simulink library "MicaServo"  (Simulink 4.00)
settings Model: LastModifiedBy=Administrator

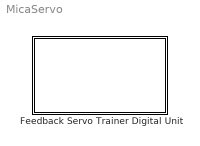
== system MicaServo ==
  Feedback Servo Trainer Digital Unit : Subsystem
      settings: RTWFcnNameOpts=Auto  RTWFileNameOpts=Auto
      mask Type: Feedback Servo Trainer Digital Unit with Mica926
      mask Display: disp ('Feedback 33-003 \n\n Digital Servo Fundementals \n with MICA 926')

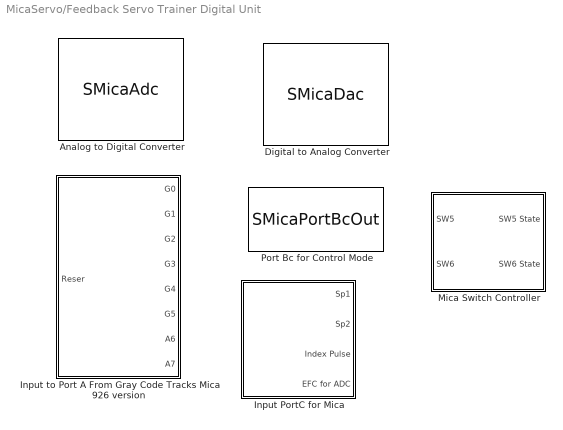
== system MicaServo/Feedback Servo Trainer Digital Unit ==
  " Digital to Analog Converter" : S-Function  FunctionName=SMicaDac  Parameters=baseAddr,inType,stime,hwAccess  PortCounts=[]  SFunctionModules=''  mask( Digital to Analog Converter){baseAddr=0x300, inType=RawData (-127 to +127), stime=0.01, hwAccess=on}
      mask prompts: baseAddr "BaseAddress"; inType "Input Type"; stime "Sampling Time (sec.)"; hwAccess "Access Hardware"
      mask help:
      | Analog Input Unit for Feedback DU154B
      | Digital Unit 33-003
      | Feeback Instruments
      | MICA 926 Edition
      mask Help:
      | Applies the corresponding voltage to the Servo Trainers DAC
      | output type can be selected to be either in RawData type or directly in volts
      mask StyleString: edit,popup(RawData (-127 to +127)| Volt   (+/- 11V range)),edit,checkbox
      mask Display: disp('Feedback Servo Trainer\n Digital Unit 33-003\n\n DAC\n Mica 926 Board ')
  Analog to Digital Converter : S-Function  FunctionName=SMicaAdc  Parameters=baseAddr,inType,stime,hwAccess  PortCounts=[]  SFunctionModules=''  mask(Analog to Digital Converter){baseAddr=0x300, inType=RawData (-127 to +127), stime=0.01, hwAccess=on}
      mask prompts: baseAddr "BaseAddress"; inType "Input Type"; stime "Sampling Time (sec.)"; hwAccess "Access Hardware"
      mask help:
      | Analog Input Unit for Feedback DU154B
      | Digital Unit 33-003
      | Feeback Instruments
      mask Help:
      | Reads and converts the voltage applied to ADC input on the Digital Unit.
      | Read operation is done either in Rawdata (+/- 127) format or directly in voltage format
      mask StyleString: edit,popup(RawData (-127 to +127)| Volt   (+/- 11V range)),edit,checkbox
      mask Display: disp('Feedback Servo Trainer\n Digital Unit 33-003\n\n ADC\n Mica 926 Board ')
  Input PortC for Mica : Subsystem  mask(Read the Inputs from portC directly){baseAddr=0x300, stime=0.01, hwAccess=on}
      mask prompts: baseAddr "BaseAddress"; stime "Sample Time (sec.)"; hwAccess "Access Hardware"
      settings: RTWFcnNameOpts=Auto  RTWFileNameOpts=Auto
  Input to Port A From Gray Code Tracks Mica 926 version : Subsystem  mask(Read Gray Code and Speed Tracks){baseAddr=0x300, stime=0.01, hwAccess=on}
      mask prompts: baseAddr "BaseAddress"; stime "Sample Time (sec.)"; hwAccess "Hardware Access"
      mask help:
      | Read the inputs from the Gray Code tracks (A0-A5)
      | and Speed/Increment tracks (A6-A7)
      settings: RTWFcnNameOpts=Auto  RTWFileNameOpts=Auto
      mask Help: no help is available for this block
  Mica Switch Controller : Subsystem  mask(Mica Switch Controller){baseAddr=0x300, onWhen=1.0, stime=0.01, hwAccess=on}
      mask prompts: baseAddr "BaseAddress"; onWhen "Thresh Hold"; stime "Sample Time (sec.)"; hwAccess "Hardware Access"
      mask help:
      | Controls the SW5 and SW6 switches on the Digital Unit
      | The ouptut can be used to see the state of the switches
      settings: RTWFcnNameOpts=Auto  RTWFileNameOpts=Auto
      mask Help: The Switches will be on when the input to the Swiches are bigger than or equal to the "Thresh Hold" variable
  Port Bc for Control Mode : S-Function  FunctionName=SMicaPortBcOut  Parameters=baseAddr,stime,hwAccess  PortCounts=[]  SFunctionModules=''  mask(Port Bc for Direct access to Control Signals){baseAddr=0x300, stime=0.01, hwAccess=on}
      mask prompts: baseAddr "Base Address"; stime "Sample Time (sec.)"; hwAccess "Access Hardware"
      mask help:
      | To directly access the Bc control register
      | For Advanced users only !
      mask Help:
      | Will directly apply the integer input to the Bc control output
      | This module is for advenced users only .
      | using this module with other Servo Trainer modules may corrupt inputs !
      mask Display: disp('Feedback Servo Trainer\n Digital Unit 33-003\n\nPort Bc \n Mica 926 Version')

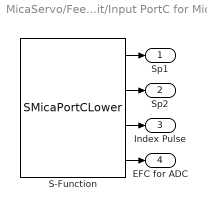
== system MicaServo/Feedback Servo Trainer Digital Unit/Input PortC for Mica ==
  S-Function : S-Function  FunctionName=SMicaPortCLower  Parameters=baseAddr,stime,hwAccess  PortCounts=[]  SFunctionModules=''
  Sp1 : Outport  Port=1
  Sp2 : Outport  Port=2
  Index Pulse : Outport  Port=3
  "EFC for ADC  " : Outport  Port=4
  wires:
  S-Function/4 -> "EFC for ADC  "/1
  S-Function/3 -> Index Pulse/1
  S-Function/2 -> Sp2/1
  S-Function/1 -> Sp1/1

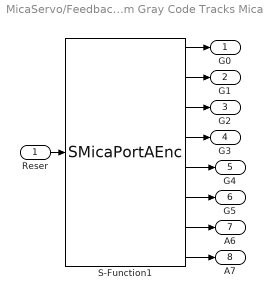
== system MicaServo/Feedback Servo Trainer Digital Unit/Input to Port A From Gray Code Tracks Mica 926 version ==
  Reser : Inport  Port=1
  S-Function1 : S-Function  FunctionName=SMicaPortAEnc  Parameters=baseAddr,stime,hwAccess  PortCounts=[]  SFunctionModules=''
  G0 : Outport  Port=1
  G1 : Outport  Port=2
  G2 : Outport  Port=3
  G3 : Outport  Port=4
  G4 : Outport  Port=5
  G5 : Outport  Port=6
  A6 : Outport  Port=7
  A7 : Outport  Port=8
  wires:
  S-Function1/8 -> A7/1
  S-Function1/7 -> A6/1
  S-Function1/6 -> G5/1
  S-Function1/5 -> G4/1
  Reser/1 -> S-Function1/1
  S-Function1/4 -> G3/1
  S-Function1/3 -> G2/1
  S-Function1/2 -> G1/1
  S-Function1/1 -> G0/1

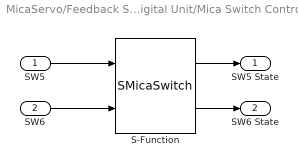
== system MicaServo/Feedback Servo Trainer Digital Unit/Mica Switch Controller ==
  SW5 : Inport  Port=1
  SW6 : Inport  Port=2
  S-Function : S-Function  FunctionName=SMicaSwitch  Parameters=baseAddr,onWhen,stime,hwAccess  PortCounts=[]  SFunctionModules=''
  SW5 State : Outport  Port=1
  SW6 State : Outport  Port=2
  wires:
  SW6/1 -> S-Function/2
  S-Function/2 -> SW6 State/1
  SW5/1 -> S-Function/1
  S-Function/1 -> SW5 State/1
